simulink model "openloop12"  (Simulink 7.5)
settings: Solver=ode45  StartTime=0.0  StopTime=5  RelTol=1e-3
undefined symbols (not defined in the file or in its folder): denz, numz
settings Model: Creator=Prof. Mahdi Mahfouf  LastModifiedBy=Prof. Mahdi Mahfouf

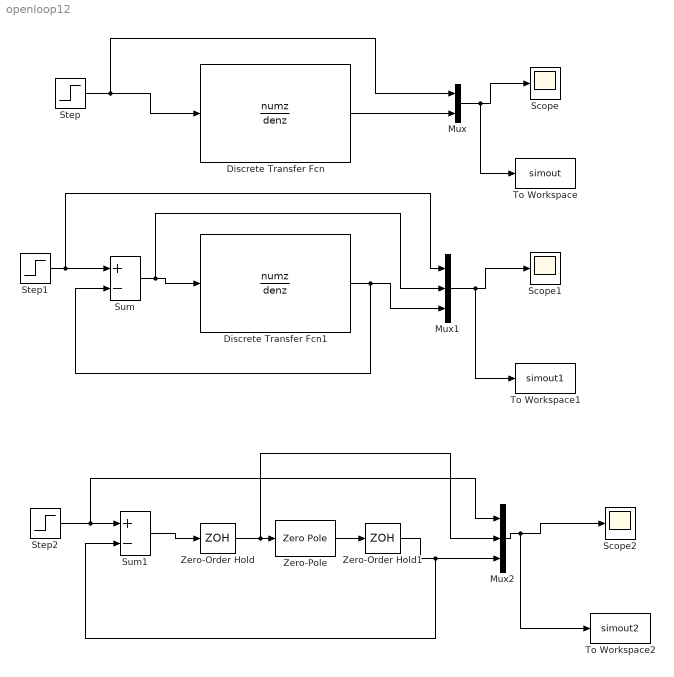
== system openloop12 ==
  Discrete Transfer Fcn : DiscreteTransferFcn  Numerator=numz  Denominator=denz  SampleTime=0.1541
  Discrete Transfer Fcn1 : DiscreteTransferFcn  Numerator=numz  Denominator=denz  SampleTime=0.1541
  Mux : Mux  Inputs=2
  Mux1 : Mux  Inputs=3
  Mux2 : Mux  Inputs=3
  Scope : Scope
  Scope1 : Scope
  Scope2 : Scope
      settings: SaveName=ScopeData2
  Step : Step  Time=0  SampleTime=0
  Step1 : Step  Time=0  SampleTime=0
  Step2 : Step  Time=0  SampleTime=0
  Sum : Sum  Inputs=+-  OutDataType=fixdt(1, 16)  OutScaling=2^0
  Sum1 : Sum  Inputs=+-  OutDataType=fixdt(1, 16)  OutScaling=2^0
  To Workspace : ToWorkspace  VariableName=simout  SampleTime=-1  SaveFormat=Structure
  To Workspace1 : ToWorkspace  VariableName=simout1  SampleTime=-1  SaveFormat=Structure
  To Workspace2 : ToWorkspace  VariableName=simout2  SampleTime=-1  SaveFormat=Structure
  Zero-Order Hold : ZeroOrderHold  SampleTime=0.1541
  Zero-Order Hold1 : ZeroOrderHold  SampleTime=0.1541
  Zero-Pole : ZeroPole  Zeros=-1  Poles=[-3 -5]
  wires:
  Step/1 -> Discrete Transfer Fcn/1, Mux/1
  Discrete Transfer Fcn/1 -> Mux/2
  Mux/1 -> Scope/1, To Workspace/1
  Step1/1 -> Sum/1, Mux1/1
  Sum/1 -> Discrete Transfer Fcn1/1, Mux1/2
  Discrete Transfer Fcn1/1 -> Mux1/3, Sum/2
  Mux1/1 -> Scope1/1, To Workspace1/1
  Step2/1 -> Sum1/1, Mux2/1
  Sum1/1 -> Zero-Order Hold/1
  Zero-Order Hold/1 -> Zero-Pole/1, Mux2/2
  Zero-Pole/1 -> Zero-Order Hold1/1
  Zero-Order Hold1/1 -> Mux2/3, Sum1/2
  Mux2/1 -> Scope2/1, To Workspace2/1
